simulink model "pathProjectionNumerical_th"  (R2018b)
settings: Solver=FixedStepAuto  StartTime=0.0  StopTime=0.001  FixedStep=0.001  RelTol=1e-3
values from neighbouring files (symbols this model uses):
  positionX_m = 0.072905510368239    (= 0.0729055103682)    [pathProjectionNumerical_ts.m]
  positionY_m = 0.150971219010512    (= 0.150971219011)    [pathProjectionNumerical_ts.m]
  previousPathPosition = 3.599999999999159e-04    (= 0.00036)    [pathProjectionNumerical_ts.m]
libraries: pathProjectionNumerical_ul x1
settings Model: Creator=mcobb  LastModifiedBy=mitch
settings DebuggingCC: LibraryContextMissingDiagnostic=none
settings SFSimCC: SimUseLocalCustomCode=off
settings RTWCC: RTWUseLocalCustomCode=off

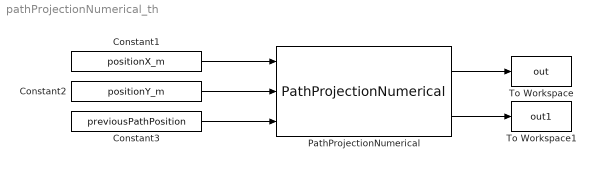
== system pathProjectionNumerical_th ==
  Constant1 : Constant  Value=positionX_m
  Constant2 : Constant  Value=positionY_m
  Constant3 : Constant  Value=previousPathPosition
  PathProjectionNumerical : pathProjectionNumerical_ul/PathProjectionNumerical  sDist=searchDistance_none  brkpts=projectionBreakpoints  xVals=projectionX  yVals=projectionY
  To Workspace : ToWorkspace  VariableName=out  SaveFormat=Timeseries  SampleTime=-1
  To Workspace1 : ToWorkspace  VariableName=out1  SaveFormat=Timeseries  SampleTime=-1
  wires:
  PathProjectionNumerical/1 -> To Workspace/1
  Constant1/1 -> PathProjectionNumerical/1
  Constant2/1 -> PathProjectionNumerical/2
  Constant3/1 -> PathProjectionNumerical/3
  PathProjectionNumerical/2 -> To Workspace1/1
